simulink model "SVPWM_model"  (R2023b)
settings: Solver=VariableStepAuto  StartTime=0.0  StopTime=1  MaxStep=0.0001  RelTol=1e-3
libraries: spsMosfetLib x6, spsDCVoltageSourceLib x1, spsGroundLib x1, spsTriangleGeneratorLib x1, spsThreePhaseSeriesRLCBranchLib x1, spsThreePhaseVIMeasurementLib x1, sps_lib x1
settings Model: Creator=oscar  LastModifiedBy=oscar

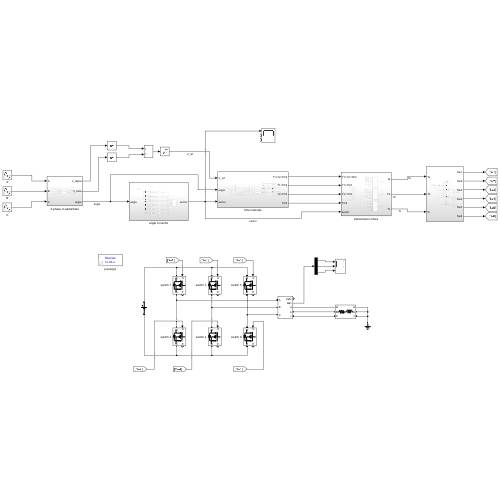
[thumbnail: Simulink's stored preview of the top-level diagram]
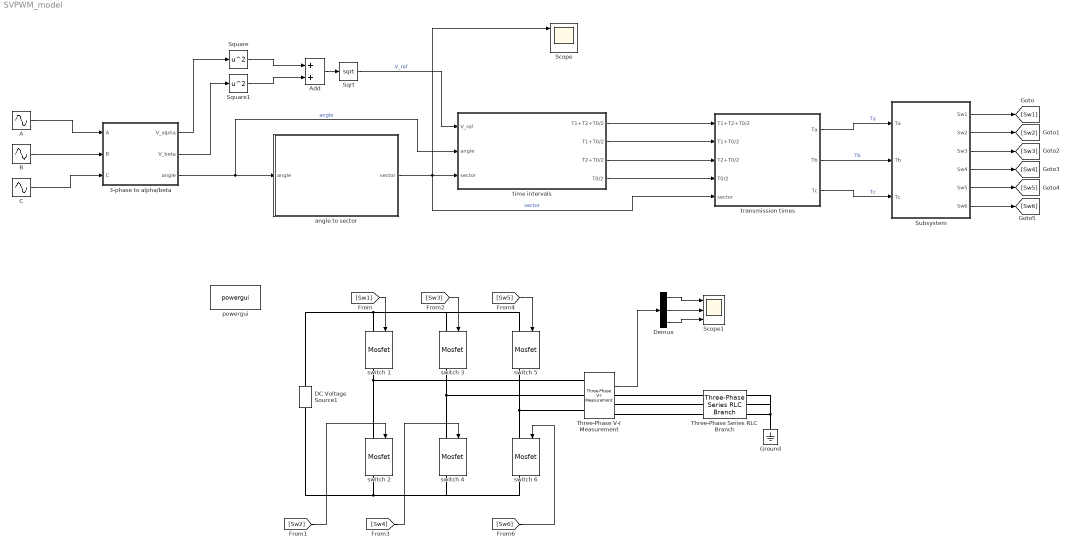
== system SVPWM_model ==
  3-phase to alpha/beta : Subsystem
  A : Sin  Frequency=2*pi*50  SampleTime=0
  Add : Sum
  B : Sin  Frequency=2*pi*50  Phase=2*pi/3  SampleTime=0
  C : Sin  Frequency=2*pi*50  Phase=4*pi/3  SampleTime=0
  DC Voltage Source1 : spsDCVoltageSourceLib/DC Voltage Source  Amplitude=100  Measurements=None
  Demux : Demux  Outputs=3
  Ground : spsGroundLib/Ground  LConnTagsString=a
  Scope : Scope  NumInputPorts=3
  Scope1 : Scope  NumInputPorts=3
  Sqrt : Sqrt
  Square : Math  Operator=square
  Square1 : Math  Operator=square
  Subsystem : Subsystem
  Three-Phase Series RLC Branch : spsThreePhaseSeriesRLCBranchLib/Three-Phase Series RLC Branch  LConnTagsString=A|B|C  RConnTagsString=A|B|C  BranchType=RL  Resistance=1  Inductance=1e-3  Capacitance=1e-6  Measurements=None
  Three-Phase V-I Measurement : spsThreePhaseVIMeasurementLib/Three-Phase V-I Measurement  VoltageMeasurement=phase-to-ground  SetLabelV=off  LabelV=Vabc  Vpu=off  VpuLL=off  CurrentMeasurement=yes  SetLabelI=off  LabelI=Iabc  Ipu=off  Pbase=100e6  Vbase=500e3  OutputType=Complex  PhasorSimulation=off  PSBequivalent=0
  angle to sector : Subsystem
  powergui : sps_lib/powergui  Priority=1  SimulationMode=Discrete  SampleTime=1e-6  frequency=60  Iterations=50  frequencyindice=0  Pbase=100e6  ErrMax=1e-4  UnitsV=kV  UnitsW=MW  buscounter=0  FunctionMessages=off  echomessages=off  EnableUseOfTLC=off  CurrentSourceSwitches=off  DisableSnubberDevices=off  DisableRonSwitches=off  DisableVfSwitches=off  DisplayEquations=off  AutomaticDiscreteSolvers=off  SolverType=Tustin/Backward Euler (TBE)  Interpol=off  ExternalGateDelay=off  methode=off  Ts=100  x0status=blocks  SPID=on  SwTol=0  HookPort=off  NonlinearTolerance=1e-4  nMaxIteration=100  ContinueOnMaxIteration=off  RestoreLinks=warning  ResistiveCurrentMeasurement=off  Frange=[0:2:500]  Ylog=off  Xlog=on  ShowGrid=off  save=off  variable=ZData  structure=0  ZoomFFT=off  StartTime=0.0  cycles=1  DisplayStyle=1  fundamental=60  FreqAxis=off  MaxFrequency=1000  frequencyindicesteady=1  RmsSteady=1  display=off
  switch {1..6} (6 alike) : spsMosfetLib/Mosfet  Ron=0.1  Lon=0  Rd=0.01  Vfd=0  IC=0  Rs=1e5  Cs=inf  Measurements=on
  time intervals : Subsystem
  transmission times : Subsystem
  wires:
  A/1 -> 3-phase to alpha/beta/1(A)
  B/1 -> 3-phase to alpha/beta/2(B)
  C/1 -> 3-phase to alpha/beta/3(C)
  3-phase to alpha/beta/1(V_alpha) -> Square/1
  3-phase to alpha/beta/2(V_beta) -> Square1/1
  3-phase to alpha/beta/3(angle) -> time intervals/2(angle), angle to sector/1(angle)  "angle"
  angle to sector/1(sector) -> time intervals/3(sector), transmission times/5(sector), Scope/1  "sector"
  time intervals/1(T1+T2+T0/2) -> transmission times/1(T1+T2+T0/2)
  time intervals/2(T1+T0/2) -> transmission times/2(T1+T0/2)
  time intervals/3(T2+T0/2) -> transmission times/3(T2+T0/2)
  time intervals/4(T0/2) -> transmission times/4(T0/2)
  transmission times/2(Tb) -> Subsystem/2(Tb)  "Tb"
  transmission times/1(Ta) -> Subsystem/1(Ta)  "Ta"
  transmission times/3(Tc) -> Subsystem/3(Tc)  "Tc"
  Add/1 -> Sqrt/1
  Square/1 -> Add/1
  Square1/1 -> Add/2
  Sqrt/1 -> time intervals/1(V_ref)  "V_ref"
  [Sw1] -> switch 1/1
  [Sw2] -> switch 2/1
  [Sw3] -> switch 3/1
  [Sw4] -> switch 4/1
  [Sw5] -> switch 5/1
  [Sw6] -> switch 6/1
  Subsystem/1(Sw1) -> [Sw1]
  Subsystem/2(Sw2) -> [Sw2]
  Subsystem/3(Sw3) -> [Sw3]
  Subsystem/4(Sw4) -> [Sw4]
  Subsystem/5(Sw5) -> [Sw5]
  Subsystem/6(Sw6) -> [Sw6]
  Demux/1 -> Scope1/1
  Demux/3 -> Scope1/3
  Demux/2 -> Scope1/2
  Three-Phase V-I Measurement/2 -> Demux/1
  connections:
  DC Voltage Source1/LConn1 -- switch 6/RConn1 -- switch 4/RConn1 -- switch 2/RConn1
  DC Voltage Source1/RConn1 -- switch 1/LConn1 -- switch 3/LConn1 -- switch 5/LConn1
  switch 1/RConn1 -- Three-Phase V-I Measurement/LConn1 -- switch 2/LConn1
  switch 5/RConn1 -- Three-Phase V-I Measurement/LConn3 -- switch 6/LConn1
  switch 3/RConn1 -- Three-Phase V-I Measurement/LConn2 -- switch 4/LConn1
  Three-Phase Series RLC Branch/LConn1 -- Three-Phase V-I Measurement/RConn1
  Three-Phase Series RLC Branch/LConn2 -- Three-Phase V-I Measurement/RConn2
  Three-Phase Series RLC Branch/LConn3 -- Three-Phase V-I Measurement/RConn3
  Ground/LConn1 -- Three-Phase Series RLC Branch/RConn1 -- Three-Phase Series RLC Branch/RConn2 -- Three-Phase Series RLC Branch/RConn3

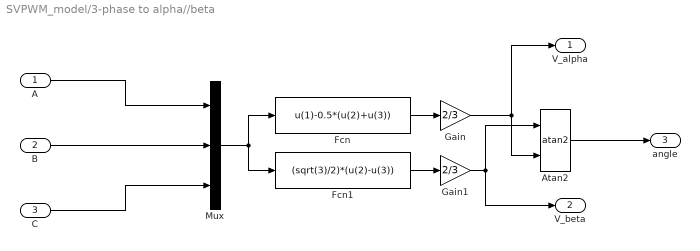
== system SVPWM_model/3-phase to alpha//beta ==
  A : Inport
  B : Inport  Port=2
  C : Inport  Port=3
  Atan2 : Trigonometry  Operator=atan2
  Fcn : Fcn  Expr=u(1)-0.5*(u(2)+u(3))
  Fcn1 : Fcn  Expr=(sqrt(3)/2)*(u(2)-u(3))
  Gain : Gain  Gain=2/3
  Gain1 : Gain  Gain=2/3
  Mux : Mux  Inputs=3
  V_alpha : Outport
  V_beta : Outport  Port=2
  angle : Outport  Port=3
  wires:
  Fcn1/1 -> Gain1/1
  Gain1/1 -> V_beta/1, Atan2/1
  Gain/1 -> V_alpha/1, Atan2/2
  Atan2/1 -> angle/1
  A/1 -> Mux/1
  Mux/1 -> Fcn1/1, Fcn/1
  B/1 -> Mux/2
  Fcn/1 -> Gain/1
  C/1 -> Mux/3

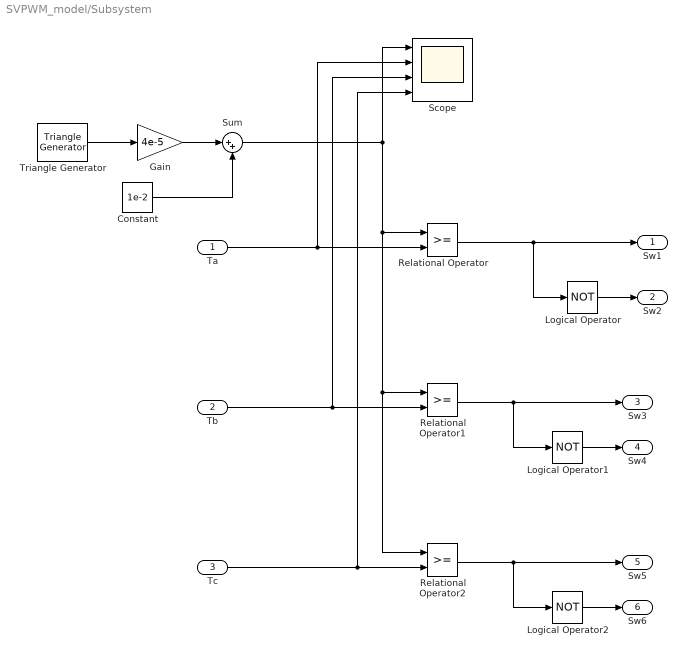
== system SVPWM_model/Subsystem ==
  Ta : Inport
  Tb : Inport  Port=2
  Tc : Inport  Port=3
  Constant : Constant  Value=1e-2
  Gain : Gain  Gain=4e-5
  Logical Operator : Logic  Operator=NOT  AllPortsSameDT=off  OutDataTypeStr=boolean
  Logical Operator1 : Logic  Operator=NOT  AllPortsSameDT=off  OutDataTypeStr=boolean
  Logical Operator2 : Logic  Operator=NOT  AllPortsSameDT=off  OutDataTypeStr=boolean
  Relational Operator : RelationalOperator  OutDataTypeStr=boolean  RndMeth=Simplest  InputSameDT=off
  Relational Operator1 : RelationalOperator  OutDataTypeStr=boolean  RndMeth=Simplest  InputSameDT=off
  Relational Operator2 : RelationalOperator  OutDataTypeStr=boolean  RndMeth=Simplest  InputSameDT=off
  Scope : Scope  NumInputPorts=4
  Sum : Sum  Inputs=|++
  Triangle Generator : spsTriangleGeneratorLib/Triangle Generator  Freq=10e3  Phase=90  Ts=0
  Sw1 : Outport
  Sw2 : Outport  Port=2
  Sw3 : Outport  Port=3
  Sw4 : Outport  Port=4
  Sw5 : Outport  Port=5
  Sw6 : Outport  Port=6
  wires:
  Relational Operator/1 -> Sw1/1, Logical Operator/1
  Ta/1 -> Relational Operator/2, Scope/2
  Relational Operator1/1 -> Sw3/1, Logical Operator1/1
  Tb/1 -> Relational Operator1/2, Scope/3
  Tc/1 -> Relational Operator2/2, Scope/4
  Relational Operator2/1 -> Sw5/1, Logical Operator2/1
  Logical Operator/1 -> Sw2/1
  Logical Operator2/1 -> Sw6/1
  Logical Operator1/1 -> Sw4/1
  Sum/1 -> Scope/1, Relational Operator/1, Relational Operator2/1, Relational Operator1/1
  Triangle Generator/1 -> Gain/1
  Gain/1 -> Sum/1
  Constant/1 -> Sum/2

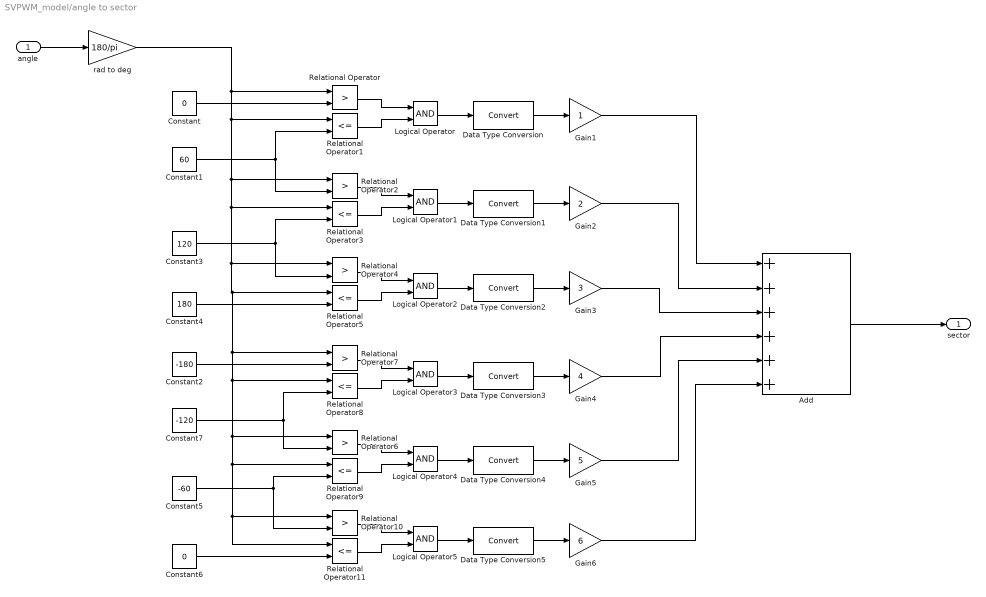
== system SVPWM_model/angle to sector ==
  angle : Inport
  Add : Sum  Inputs=++++++
  Constant : Constant  Value=0
  Constant1 : Constant  Value=60
  Constant2 : Constant  Value=-180
  Constant3 : Constant  Value=120
  Constant4 : Constant  Value=180
  Constant5 : Constant  Value=-60
  Constant6 : Constant  Value=0
  Constant7 : Constant  Value=-120
  Data Type Conversion{,1..5} (6 alike) : DataTypeConversion  SaturateOnIntegerOverflow=off  RndMeth=Floor
  Gain1 : Gain
  Gain2 : Gain  Gain=2
  Gain3 : Gain  Gain=3
  Gain4 : Gain  Gain=4
  Gain5 : Gain  Gain=5
  Gain6 : Gain  Gain=6
  Logical Operator{,1..5} (6 alike) : Logic  AllPortsSameDT=off  OutDataTypeStr=boolean
  Relational Operator{,2,4,6..7,10} (6 alike) : RelationalOperator  Operator=>  OutDataTypeStr=boolean  RndMeth=Simplest  InputSameDT=off
  Relational Operator{1,3,5,8..9,11} (6 alike) : RelationalOperator  Operator=<=  OutDataTypeStr=boolean  RndMeth=Simplest  InputSameDT=off
  rad to deg : Gain  Gain=180/pi
  sector : Outport
  wires:
  Logical Operator1/1 -> Data Type Conversion1/1
  Relational Operator10/1 -> Logical Operator5/1
  Data Type Conversion/1 -> Gain1/1
  Constant5/1 -> Relational Operator9/2, Relational Operator10/2
  Relational Operator9/1 -> Logical Operator4/2
  Relational Operator8/1 -> Logical Operator3/2
  rad to deg/1 -> Relational Operator/1, Relational Operator5/1, Relational Operator11/1, Relational Operator10/1, Relational Operator9/1, Relational Operator6/1, Relational Operator8/1, Relational Operator7/1, Relational Operator4/1, Relational Operator3/1, Relational Operator2/1, Relational Operator1/1
  Relational Operator1/1 -> Logical Operator/2
  Constant1/1 -> Relational Operator2/2, Relational Operator1/2
  Relational Operator7/1 -> Logical Operator3/1
  Constant3/1 -> Relational Operator3/2, Relational Operator4/2
  Relational Operator6/1 -> Logical Operator4/1
  Logical Operator5/1 -> Data Type Conversion5/1
  Logical Operator4/1 -> Data Type Conversion4/1
  Constant7/1 -> Relational Operator8/2, Relational Operator6/2
  angle/1 -> rad to deg/1
  Constant2/1 -> Relational Operator7/2
  Data Type Conversion1/1 -> Gain2/1
  Gain2/1 -> Add/2
  Add/1 -> sector/1
  Relational Operator2/1 -> Logical Operator1/1
  Gain4/1 -> Add/4
  Gain6/1 -> Add/6
  Logical Operator/1 -> Data Type Conversion/1
  Relational Operator4/1 -> Logical Operator2/1
  Constant4/1 -> Relational Operator5/2
  Relational Operator11/1 -> Logical Operator5/2
  Data Type Conversion3/1 -> Gain4/1
  Relational Operator5/1 -> Logical Operator2/2
  Logical Operator2/1 -> Data Type Conversion2/1
  Relational Operator/1 -> Logical Operator/1
  Data Type Conversion4/1 -> Gain5/1
  Data Type Conversion5/1 -> Gain6/1
  Constant/1 -> Relational Operator/2
  Relational Operator3/1 -> Logical Operator1/2
  Data Type Conversion2/1 -> Gain3/1
  Constant6/1 -> Relational Operator11/2
  Logical Operator3/1 -> Data Type Conversion3/1
  Gain1/1 -> Add/1
  Gain3/1 -> Add/3
  Gain5/1 -> Add/5

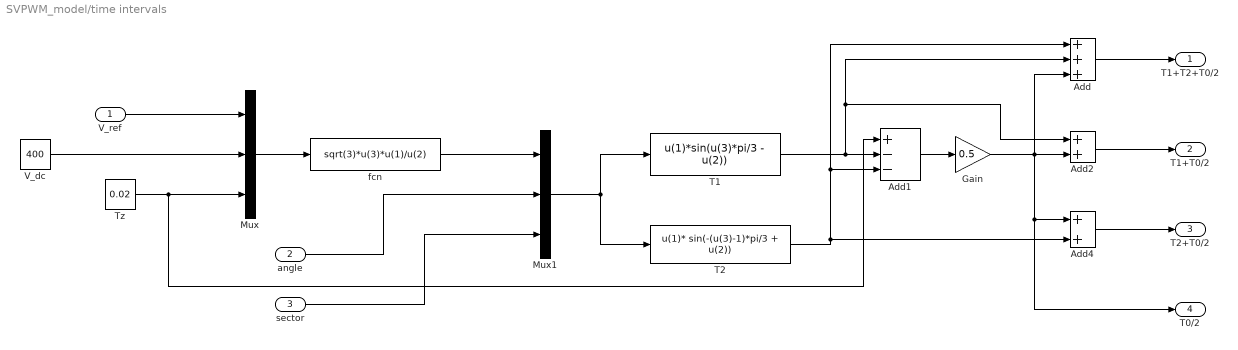
== system SVPWM_model/time intervals ==
  V_ref : Inport
  angle : Inport  Port=2
  sector : Inport  Port=3
  Add : Sum  Inputs=+++
  Add1 : Sum  Inputs=+--
  Add2 : Sum
  Add4 : Sum
  Gain : Gain  Gain=0.5
  Mux : Mux  Inputs=3
  Mux1 : Mux  Inputs=3
  T1 : Fcn  Expr=u(1)*sin(u(3)*pi/3 - u(2))
  T2 : Fcn  Expr=u(1)* sin(-(u(3)-1)*pi/3 + u(2))
  Tz : Constant  Value=0.02
  V_dc : Constant  Value=400
  fcn : Fcn  Expr=sqrt(3)*u(3)*u(1)/u(2)
  T1+T2+T0/2 : Outport
  T1+T0/2 : Outport  Port=2
  T2+T0/2 : Outport  Port=3
  T0/2 : Outport  Port=4
  wires:
  V_dc/1 -> Mux/2
  Tz/1 -> Add1/1, Mux/3
  Mux/1 -> fcn/1
  fcn/1 -> Mux1/1
  angle/1 -> Mux1/2
  sector/1 -> Mux1/3
  Mux1/1 -> T1/1, T2/1
  T1/1 -> Add/2, Add2/1, Add1/2
  T2/1 -> Add/1, Add1/3, Add4/2
  Add/1 -> T1+T2+T0/2/1
  Add1/1 -> Gain/1
  Add2/1 -> T1+T0/2/1
  Add4/1 -> T2+T0/2/1
  Gain/1 -> Add/3, Add4/1, T0/2/1, Add2/2
  V_ref/1 -> Mux/1

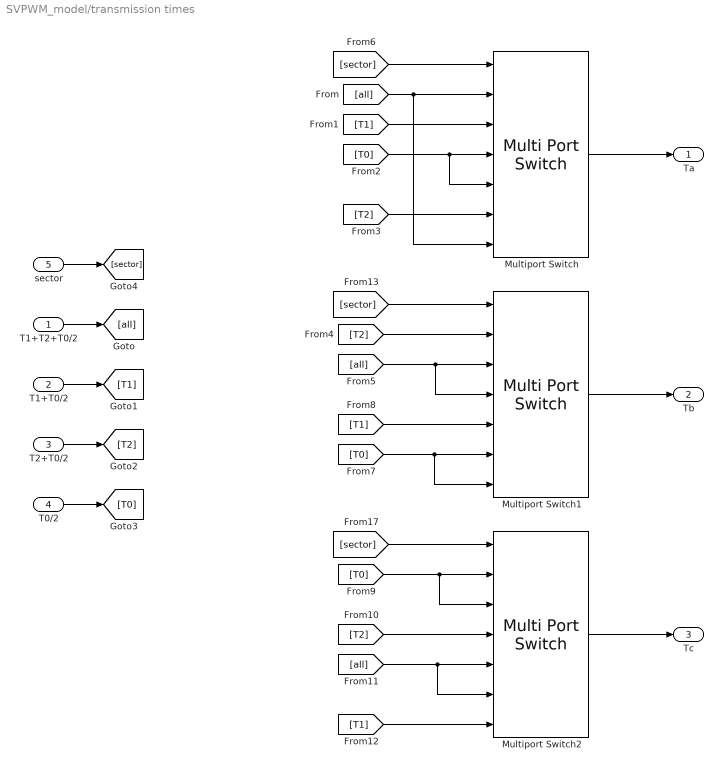
== system SVPWM_model/transmission times ==
  T1+T2+T0/2 : Inport
  T1+T0/2 : Inport  Port=2
  T2+T0/2 : Inport  Port=3
  T0/2 : Inport  Port=4
  sector : Inport  Port=5
  Multiport Switch : MultiPortSwitch  Inputs=6  DiagnosticForDefault=Warning  SaturateOnIntegerOverflow=off  InputSameDT=off
  Multiport Switch1 : MultiPortSwitch  Inputs=6  DiagnosticForDefault=Warning  SaturateOnIntegerOverflow=off  InputSameDT=off
  Multiport Switch2 : MultiPortSwitch  Inputs=6  DiagnosticForDefault=Warning  SaturateOnIntegerOverflow=off  InputSameDT=off
  Ta : Outport
  Tb : Outport  Port=2
  Tc : Outport  Port=3
  wires:
  Multiport Switch/1 -> Ta/1
  T1+T2+T0/2/1 -> [all]
  T1+T0/2/1 -> [T1]
  T2+T0/2/1 -> [T2]
  T0/2/1 -> [T0]
  sector/1 -> [sector]
  [T1] -> Multiport Switch/3
  [T0] -> Multiport Switch/5, Multiport Switch/4
  [T2] -> Multiport Switch/6
  [all] -> Multiport Switch/7, Multiport Switch/2
  [sector] -> Multiport Switch/1
  [T0] -> Multiport Switch1/7, Multiport Switch1/6
  [T2] -> Multiport Switch1/2
  [all] -> Multiport Switch1/4, Multiport Switch1/3
  [sector] -> Multiport Switch1/1
  [T1] -> Multiport Switch1/5
  Multiport Switch1/1 -> Tb/1
  [all] -> Multiport Switch2/6, Multiport Switch2/5
  Multiport Switch2/1 -> Tc/1
  [T1] -> Multiport Switch2/7
  [sector] -> Multiport Switch2/1
  [T0] -> Multiport Switch2/3, Multiport Switch2/2
  [T2] -> Multiport Switch2/4
